simulink model "zad9disc_lin"  (R2014b)
settings: Solver=ode45  StartTime=0.0  StopTime=60  RelTol=1e-3
values from neighbouring files (symbols this model uses):
  a1 = -0.28    [set_params.m]
  a2 = -0.9    [set_params.m]
  a3 = 0.35    [set_params.m]
  a4 = 0.3    [set_params.m]
  K = 4.5    [set_params.m]
  selector = 0    [zad9.m]
  T1 = 5    [set_params.m]
  T2 = 8    [set_params.m]
  Tp = 1    [zad11.m]    (also in zad3.m = Tp_vect(i); zad9.m)
  u_lin = linspace(-1,1,101)    [zad11.m]    (also in zad12.m = 1; zad6.m = K*a1*u + K*(a2*(u_p^2) + a3*(u_p^3) + a4*(u_p^4)) + K*(u - u; zad9.m = pkt_lin(i))
libraries: simulink x2
settings Model: Creator=kuba  LastModifiedBy=kuba

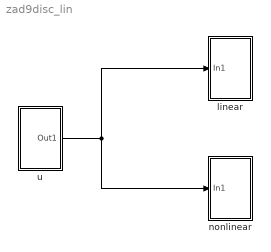
== system zad9disc_lin ==
  "linear " : Subsystem
  "nonlinear " : Subsystem
  "u " : Subsystem
  wires:
  "u "/1(Out1) -> "nonlinear "/1(In1), "linear "/1(In1)

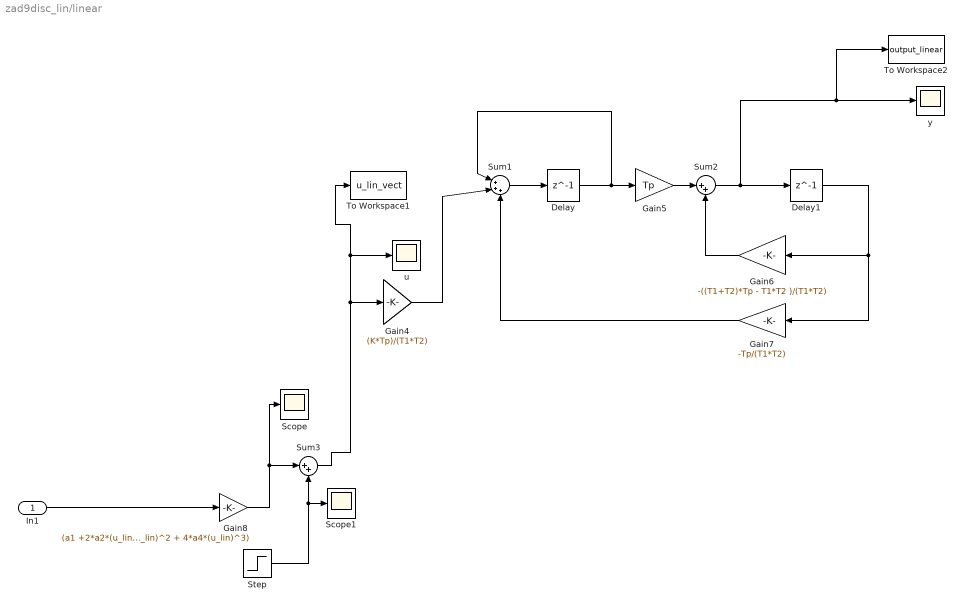
== system zad9disc_lin/linear  ==
  In1 : Inport
  Delay : Delay  DelayLength=1  SampleTime=Tp
  Delay1 : Delay  DelayLength=1  SampleTime=Tp
  Gain4 : Gain  Gain=(K*Tp)/(T1*T2)
  Gain5 : Gain  Gain=Tp
  Gain6 : Gain  Gain=-((T1+T2)*Tp - T1*T2 )/(T1*T2)
  Gain7 : Gain  Gain=-Tp/(T1*T2)
  Gain8 : Gain  Gain=(a1 +2*a2*(u_lin) + 3*a3*(u_lin)^2 + 4*a4*(u_lin)^3)  SampleTime=Tp
  Scope : Scope
      settings: SaveName=ScopeData4
  Scope1 : Scope
      settings: SaveName=ScopeData5
  Step : Step  After=-a2*(u_lin^2) -2*a3*(u_lin^3) - 3*a4*(u_lin^4)  SampleTime=0
  Sum1 : Sum  Inputs=|+++
  Sum2 : Sum  Inputs=|++
  Sum3 : Sum  Inputs=|++
  To Workspace1 : ToWorkspace  VariableName=u_lin_vect  SaveFormat=Timeseries  SampleTime=-1
  To Workspace2 : ToWorkspace  VariableName=output_linear  SaveFormat=Timeseries  SampleTime=-1
  u : Scope
  y : Scope
      settings: TimeRange=60  YMin=-2.5  YMax=0
  wires:
  Gain5/1 -> Sum2/1
  Gain4/1 -> Sum1/2
  Gain6/1 -> Sum2/2
  Gain7/1 -> Sum1/3
  Delay1/1 -> Gain7/1, Gain6/1
  Delay/1 -> Gain5/1, Sum1/1
  Sum2/1 -> To Workspace2/1, y/1, Delay1/1
  Sum1/1 -> Delay/1
  Sum3/1 -> To Workspace1/1, u/1, Gain4/1
  In1/1 -> Gain8/1
  Gain8/1 -> Scope/1, Sum3/1
  Step/1 -> Scope1/1, Sum3/2

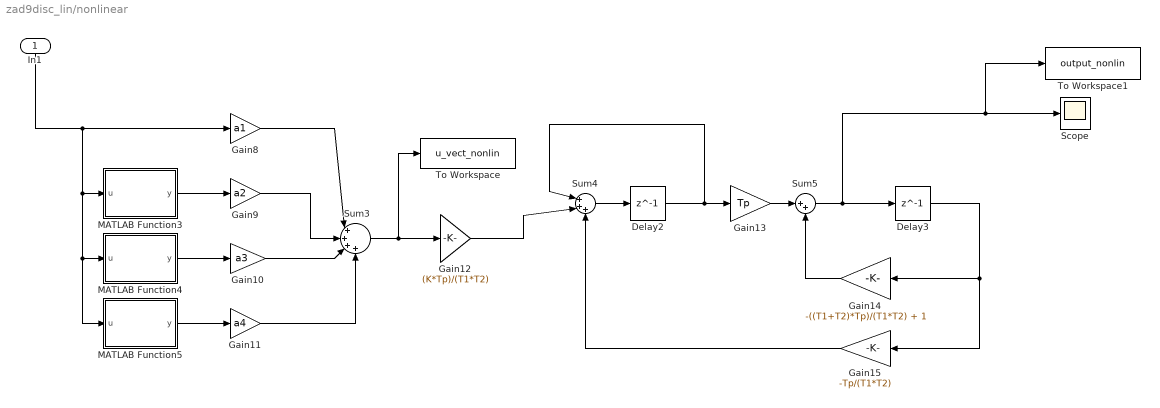
== system zad9disc_lin/nonlinear  ==
  In1 : Inport
  Delay2 : Delay  DelayLength=1  SampleTime=Tp
  Delay3 : Delay  DelayLength=1  SampleTime=Tp
  Gain10 : Gain  Gain=a3  SampleTime=Tp
  Gain11 : Gain  Gain=a4  SampleTime=Tp
  Gain12 : Gain  Gain=(K*Tp)/(T1*T2)
  Gain13 : Gain  Gain=Tp
  Gain14 : Gain  Gain=-((T1+T2)*Tp)/(T1*T2) + 1
  Gain15 : Gain  Gain=-Tp/(T1*T2)
  Gain8 : Gain  Gain=a1  SampleTime=Tp
  Gain9 : Gain  Gain=a2  SampleTime=Tp
  MATLAB Function3 : MATLAB Function  TreatAsAtomicUnit=on
  MATLAB Function4 : MATLAB Function  TreatAsAtomicUnit=on
  MATLAB Function5 : MATLAB Function  TreatAsAtomicUnit=on
  Scope : Scope
      settings: TimeRange=100  YMin=-1  YMax=1  SaveName=ScopeData3
  Sum3 : Sum  Inputs=|++++
  Sum4 : Sum  Inputs=|+++
  Sum5 : Sum  Inputs=|++
  To Workspace : ToWorkspace  VariableName=u_vect_nonlin  SaveFormat=Timeseries  SampleTime=-1
  To Workspace1 : ToWorkspace  VariableName=output_nonlin  SaveFormat=Timeseries  SampleTime=-1
  wires:
  In1/1 -> MATLAB Function5/1(u), MATLAB Function4/1(u), MATLAB Function3/1(u), Gain8/1
  Gain15/1 -> Sum4/3
  Gain10/1 -> Sum3/3
  MATLAB Function3/1(y) -> Gain9/1
  MATLAB Function4/1(y) -> Gain10/1
  Gain9/1 -> Sum3/2
  Sum3/1 -> To Workspace/1, Gain12/1
  Gain8/1 -> Sum3/1
  Gain12/1 -> Sum4/2
  Sum4/1 -> Delay2/1
  Gain13/1 -> Sum5/1
  Sum5/1 -> To Workspace1/1, Scope/1, Delay3/1
  Gain14/1 -> Sum5/2
  Delay3/1 -> Gain15/1, Gain14/1
  Gain11/1 -> Sum3/4
  Delay2/1 -> Gain13/1, Sum4/1
  MATLAB Function5/1(y) -> Gain11/1

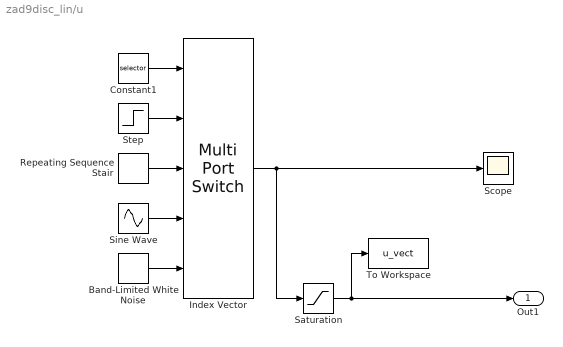
== system zad9disc_lin/u  ==
  Band-Limited White Noise : simulink/Sources/Band-Limited White Noise  Cov=[0.1]  Ts=0.1  seed=[23341]
  Constant1 : Constant  Value=selector
  Index Vector : MultiPortSwitch  DataPortOrder=Zero-based contiguous  Inputs=4  zeroidx=on
  Repeating Sequence Stair : simulink/Sources/Repeating Sequence Stair  OutValues=[0.4 0.8 1 0.4 -0.2 -0.6 -1 -0.6].'  tsamp=5  OutMin=[]  OutMax=[]  OutDataTypeStr=double  OutputDataTypeScalingMode=double  OutDataType=fixdt(0,8)  ConRadixGroup=Best Precision: Vector-wise  OutScaling=2^-12
  Saturation : Saturate  UpperLimit=1  LowerLimit=-1
  Scope : Scope
      settings: TimeRange=50  YMin=-1  YMax=1  SaveName=ScopeData2
  Sine Wave : Sin  SampleTime=0
  Step : Step  SampleTime=0
  To Workspace : ToWorkspace  VariableName=u_vect  SaveFormat=Timeseries  SampleTime=-1
  Out1 : Outport
  wires:
  Band-Limited White Noise/1 -> Index Vector/5
  Sine Wave/1 -> Index Vector/4
  Index Vector/1 -> Saturation/1, Scope/1
  Constant1/1 -> Index Vector/1
  Repeating Sequence Stair/1 -> Index Vector/3
  Saturation/1 -> To Workspace/1, Out1/1
  Step/1 -> Index Vector/2

== matlab function zad9disc_lin/nonlinear /MATLAB Function3 ==
  data: u input; y output
function y = square(u)
y = u^2;

== matlab function zad9disc_lin/nonlinear /MATLAB Function4 ==
  data: u input; y output
function y = cube(u)
y = u^3;

== matlab function zad9disc_lin/nonlinear /MATLAB Function5 ==
  data: u input; y output
function y = quad(u)
y = u^4;
